simulink model "satellite_sim"  (Simulink 7.7)
settings: Solver=ode45  StartTime=0.0  StopTime=200  RelTol=1e-3
undefined symbols (not defined in the file or in its folder): drawSatellite, P, satellite_ctrl
settings Model: Creator=beard  LastModifiedBy=beard
settings OptimizationCC: InitFltsAndDblsToZero=on
settings DebuggingCC: StrictBusMsg=Warning

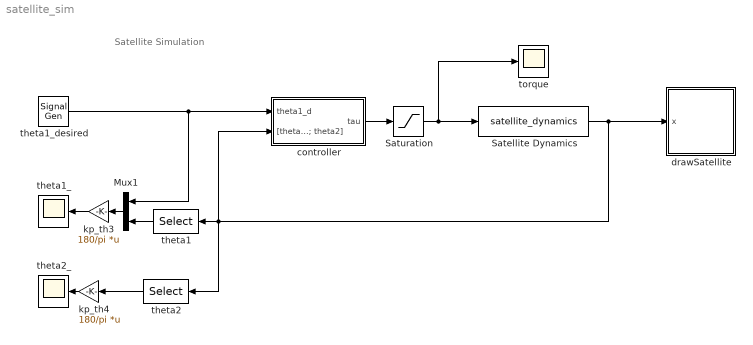
== system satellite_sim ==
  note: Satellite Simulation
  Mux1 : Mux  Inputs=2
  Satellite Dynamics : S-Function  FunctionName=satellite_dynamics  Parameters=AP  EnableBusSupport=off
  Saturation : Saturate  UpperLimit=P.tau_max  LowerLimit=-P.tau_max
  controller : Subsystem
  drawSatellite : Subsystem
      mask init:
      | % drawing parameters
      | L = 1;
      | w = .3;
      mask Display: image(imread('tv.jpg'))
  kp_th3 : Gain  Gain=180/pi  Multiplication=Matrix(K*u)
  kp_th4 : Gain  Gain=180/pi  Multiplication=Matrix(K*u)
  theta1 : Selector  InputPortWidth=2  IndexOptions=Index vector (dialog)  Indices=[1]  OutputSizes=1
  theta1_ : Scope
      settings: TimeRange=200  YMin=-22.5  YMax=22.5  SaveName=ScopeData2
  theta1_desired : SignalGenerator  WaveForm=square  Amplitude=20*pi/180  Frequency=.005
  theta2 : Selector  InputPortWidth=2  IndexOptions=Index vector (dialog)  Indices=[2]  OutputSizes=1
  theta2_ : Scope
      settings: TimeRange=200  YMin=-20  YMax=17.5
  torque : Scope
      settings: TimeRange=200  YMin=-0.7  YMax=0.4
  wires:
  Satellite Dynamics/1 -> drawSatellite/1(x), controller/2("[theta1; theta2]"), theta1/1, theta2/1
  Saturation/1 -> torque/1, Satellite Dynamics/1
  Mux1/1 -> kp_th3/1
  kp_th3/1 -> theta1_/1
  kp_th4/1 -> theta2_/1
  controller/1(tau) -> Saturation/1
  theta1_desired/1 -> controller/1(theta1_d), Mux1/1
  theta1/1 -> Mux1/2
  theta2/1 -> kp_th4/1

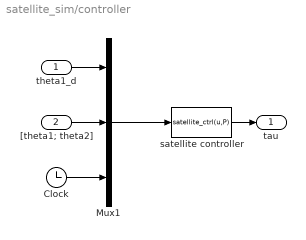
== system satellite_sim/controller ==
  theta1_d : Inport
  "[theta1; theta2]" : Inport  Port=2
  Clock : Clock
      settings: Decimation=10
  Mux1 : Mux  Inputs=3
  satellite controller : MATLABFcn  MATLABFcn=satellite_ctrl(u,P)  OutputDimensions=1  SampleTime=P.Ts
  tau : Outport
  wires:
  Clock/1 -> Mux1/3
  satellite controller/1 -> tau/1
  "[theta1; theta2]"/1 -> Mux1/2
  theta1_d/1 -> Mux1/1
  Mux1/1 -> satellite controller/1

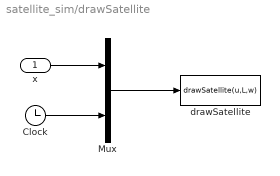
== system satellite_sim/drawSatellite ==
  x : Inport
  Clock : Clock
      settings: Decimation=10
  Mux : Mux  Inputs=2
  drawSatellite : MATLABFcn  MATLABFcn=drawSatellite(u,L,w)  OutputDimensions=0  SampleTime=0.1
  wires:
  Mux/1 -> drawSatellite/1
  x/1 -> Mux/1
  Clock/1 -> Mux/2
